simulink model "ControlUnit"  (R2025b)
settings: Solver=VariableStepAuto  StartTime=0.0  StopTime=10.0  RelTol=1e-3
settings Model: Creator=cyber  LastModifiedBy=cyber

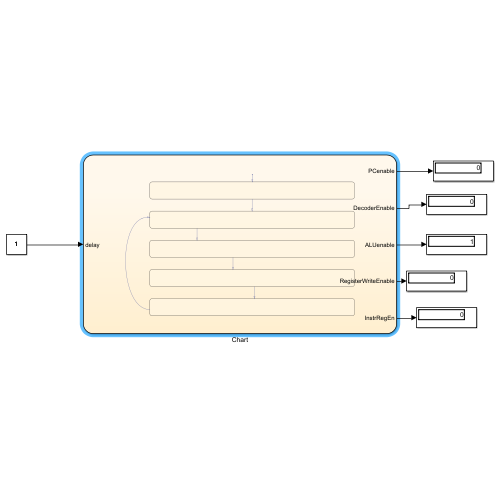
[thumbnail: Simulink's stored preview of the top-level diagram]
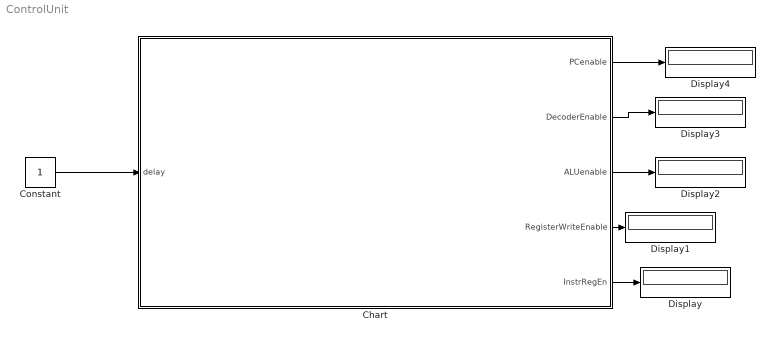
== system ControlUnit ==
  Chart : Stateflow chart  TreatAsAtomicUnit=on
  Constant : Constant
  Display{,1..4} (5 alike) : Display
  wires:
  Chart/5(InstrRegEn) -> Display/1
  Chart/4(RegisterWriteEnable) -> Display1/1
  Chart/3(ALUenable) -> Display2/1
  Chart/2(DecoderEnable) -> Display3/1
  Chart/1(PCenable) -> Display4/1
  Constant/1 -> Chart/1(delay)

== stateflow chart ControlUnit/Chart ==
  state Start
    PCenable=0;InstrRegEn=0;DecoderEnable=0;ALUenable=0;RegisterWriteEnable=0;
  state Fetch
    PCenable=1;InstrRegEn=1;DecoderEnable=0;ALUenable=0;RegisterWriteEnable=0;
  state Decode
    PCenable=0;InstrRegEn=1;DecoderEnable=1;ALUenable=0;RegisterWriteEnable=0;
  state Execute
    PCenable=0;InstrRegEn=0;DecoderEnable=0;ALUenable=1;RegisterWriteEnable=0;
  state Writeback
    PCenable=0;InstrRegEn=0;DecoderEnable=0;ALUenable=1;RegisterWriteEnable=1;
  (default) -> Start
  Start -> Fetch
  Writeback -> Fetch : [delay>40]
  Fetch -> Decode : [delay>10]
  Decode -> Execute : [delay>20]
  Execute -> Writeback : [delay>30]
  data: delay input; PCenable output; DecoderEnable output; ALUenable output; RegisterWriteEnable output; InstrRegEn output
